simulink model "SF049A_LoaMgr"  (R2013b)
settings: Solver=FixedStepDiscrete  SolverMode=SingleTasking  StartTime=0.0  StopTime=1  FixedStep=0.002  RelTol=1e-3
undefined symbols (not defined in the file): CURRMEASLOAMTGTNMASK_CNT_U08, IVTRLOAMTGTNMASK_CNT_U08, LoaCtrldShtdwn, LoaCurrMeasIdptSigNrFlt, LoaHwTqIdptSigNrFlt, LoaImdtShtdwn, LoaIvtrIdptSigNrFlt, LOAMAXSLEW_ULSPERSEC_F32, LoaMgrCurrIvtrMtgtnRate, LoaMgrCurrIvtrMtgtnSca, LoaMgrCurrIvtrMtgtnScaZeroEna, LoaMgrCurrMeasIdptSig0Resp, LoaMgrCurrMeasIdptSig1Resp, LoaMgrCurrMeasIdptSig2Resp, LoaMgrCurrMeasIdptSigFltThd, LoaMgrCurrMeasMtgtnRate, LoaMgrCurrMeasMtgtnSca, LoaMgrCurrMeasMtgtnScaZeroEna, LoaMgrFadeOutStRate, LoaMgrHwTqIdptSig0NoTqLoaResp, LoaMgrHwTqIdptSig1NoTqLoaResp, LoaMgrHwTqIdptSig2Resp, LoaMgrHwTqIdptSig4Resp, LoaMgrHwTqIdptSigFltThd, LoaMgrHwTqLoaAvlResp, LoaMgrIvtrIdptSig0Resp, LoaMgrIvtrIdptSig1Resp, LoaMgrIvtrIdptSig2Resp, LoaMgrIvtrIdptSigFltThd, LoaMgrIvtrMtgtnRate, LoaMgrIvtrMtgtnSca, LoaMgrIvtrMtgtnScaZeroEna, LoaMgrLimdStRate, LoaMgrLimdStSca, LoaMgrMotAgAvlSnsrlsResp, LoaMgrMotAgIdptSig0NoSnsrlsResp, LoaMgrMotAgIdptSig1NoSnsrlsResp, LoaMgrMotAgIdptSig2Resp, LoaMgrMotAgIdptSig3Resp, LoaMgrMotAgIdptSigFltThd, LoaMgrMotAgMtgtnRate, LoaMgrMotAgMtgtnSca, LoaMgrMotAgMtgtnScaZeroEna, LoaMotAgIdptSigNrFlt, LOASCAONE_ULS_F32, LOASCAZERO_ULS_F32, LoaSt1, LOASTIMDTSHTDWN_CNT_U08, LOASTNORM_CNT_U08, LOASTSWMTGTN_CNT_U08, MAXCURRMEASIDPTSIGALLWD_CNT_U08, MAXHWTQIDPTSIGALLWD_CNT_U08, MAXIVTRIDPTSIGALLWD_CNT_U08, MAXMOTAGMECLIDPTSIGALLWD_CNT_U08, NODEBSTEP_CNT_U16, NtcSts1, SigQlfr1
libraries: simulink x30, NxtrMin x4, NxtrMax x4, NxtrLim x2
(part 3 of 7)

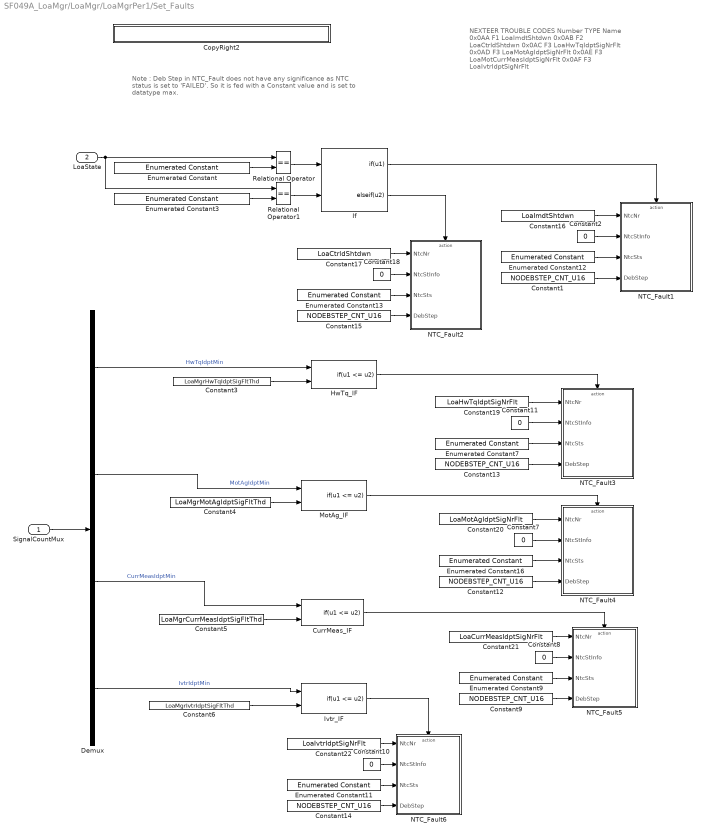
== system SF049A_LoaMgr/LoaMgr/LoaMgrPer1/Set_Faults ==
  note: Note : Deb Step in NTC_Fault does not have any significance as
      | NTC status is set to 'FAILED'. So it is fed with a Constant value and
      | is set to datatype max.
  note: NEXTEER TROUBLE CODES
      | Number  TYPE   Name
      |  0x0AA      F1      LoaImdtShtdwn
      |  0x0AB      F2      LoaCtrldShtdwn
      |  0x0AC      F3      LoaHwTqIdptSigNrFlt
      |  0x0AD      F3      LoaMotAgIdptSigNrFlt
      |  0x0AE      F3      LoaMotCurrMeasIdptSigNrFlt
      |  0x0AF      F3      LoaIvtrIdptSigNrFlt
  SignalCountMux : Inport
  LoaState : Inport  RequirementInfo={} %GIDa_be80d350_3951_4772_b695_9000f2f6daa5  Port=2
  Constant1 : Constant  RequirementInfo="{'linktype_rmi_doors' '00012fd5 (/E-STEER Core/SubSystem Specifications/Application Functions - EA4/SF049A Loss of Assist Manager)' '#SF049A_41' 'true' 'REQ:  SF049A_41' '' } %GIDa_6008ab27_f6d5_4e1f_aaef_fe9677c74400"  Value=NODEBSTEP_CNT_U16
  Constant10 : Constant  RequirementInfo="{'linktype_rmi_doors' '00012fd5 (/E-STEER Core/SubSystem Specifications/Application Functions - EA4/SF049A Loss of Assist Manager)' '#SF049A_96' 'true' 'REQ:  SF049A_96' '' } %GIDa_9d6138e1_72b7_4c86_9d87_817de0f28e02"  Value=0
  Constant11 : Constant  RequirementInfo="{'linktype_rmi_doors' '00012fd5 (/E-STEER Core/SubSystem Specifications/Application Functions - EA4/SF049A Loss of Assist Manager)' '#SF049A_63' 'true' 'REQ:  SF049A_63' '' } %GIDa_f847bbfc_c670_43d9_9c09_50e4c18d810d"  Value=0
  Constant12 : Constant  RequirementInfo="{'linktype_rmi_doors' '00012fd5 (/E-STEER Core/SubSystem Specifications/Application Functions - EA4/SF049A Loss of Assist Manager)' '#SF049A_74' 'true' 'REQ:  SF049A_74' '' } %GIDa_482641ce_f585_4632_a45d_846d40cb84bb"  Value=NODEBSTEP_CNT_U16
  Constant13 : Constant  RequirementInfo="{'linktype_rmi_doors' '00012fd5 (/E-STEER Core/SubSystem Specifications/Application Functions - EA4/SF049A Loss of Assist Manager)' '#SF049A_63' 'true' 'REQ:  SF049A_63' '' } %GIDa_516393a5_f80f_4cb2_bae9_6e4bb58c3191"  Value=NODEBSTEP_CNT_U16
  Constant14 : Constant  RequirementInfo="{'linktype_rmi_doors' '00012fd5 (/E-STEER Core/SubSystem Specifications/Application Functions - EA4/SF049A Loss of Assist Manager)' '#SF049A_96' 'true' 'REQ:  SF049A_96' '' } %GIDa_be9bb861_018d_44a6_a080_0e9c68b6dcb7"  Value=NODEBSTEP_CNT_U16
  Constant15 : Constant  RequirementInfo="{'linktype_rmi_doors' '00012fd5 (/E-STEER Core/SubSystem Specifications/Application Functions - EA4/SF049A Loss of Assist Manager)' '#SF049A_52' 'true' 'REQ:  SF049A_52' '' } %GIDa_0fe878fe_27c3_4b2a_9c4a_e08aafcb438f"  Value=NODEBSTEP_CNT_U16
  Constant16 : Constant  RequirementInfo="{'linktype_rmi_doors' '00012fd5 (/E-STEER Core/SubSystem Specifications/Application Functions - EA4/SF049A Loss of Assist Manager)' '#SF049A_41' 'true' 'REQ:  SF049A_41' '' } %GIDa_da02ad7f_2e11_4a07_a653_13476a033a59"  Value=LoaImdtShtdwn
  Constant17 : Constant  RequirementInfo="{'linktype_rmi_doors' '00012fd5 (/E-STEER Core/SubSystem Specifications/Application Functions - EA4/SF049A Loss of Assist Manager)' '#SF049A_52' 'true' 'REQ:  SF049A_52' '' } %GIDa_1c4603b7_e4a0_453d_b772_10fa4ca01a05"  Value=LoaCtrldShtdwn
  Constant18 : Constant  RequirementInfo="{'linktype_rmi_doors' '00012fd5 (/E-STEER Core/SubSystem Specifications/Application Functions - EA4/SF049A Loss of Assist Manager)' '#SF049A_52' 'true' 'REQ:  SF049A_52' '' } %GIDa_6e9baf4a_2a1d_4f2c_8c2c_bf437d4d00ad"  Value=0
  Constant19 : Constant  RequirementInfo="{'linktype_rmi_doors' '00012fd5 (/E-STEER Core/SubSystem Specifications/Application Functions - EA4/SF049A Loss of Assist Manager)' '#SF049A_63' 'true' 'REQ:  SF049A_63' '' } %GIDa_f668c260_f633_4aa9_84e3_26df089b87f3"  Value=LoaHwTqIdptSigNrFlt
  Constant2 : Constant  RequirementInfo="{'linktype_rmi_doors' '00012fd5 (/E-STEER Core/SubSystem Specifications/Application Functions - EA4/SF049A Loss of Assist Manager)' '#SF049A_41' 'true' 'REQ:  SF049A_41' '' } %GIDa_747c9c9e_ef17_47fe_b985_caf6a20fd37f"  Value=0
  Constant20 : Constant  RequirementInfo="{'linktype_rmi_doors' '00012fd5 (/E-STEER Core/SubSystem Specifications/Application Functions - EA4/SF049A Loss of Assist Manager)' '#SF049A_74' 'true' 'REQ:  SF049A_74' '' } %GIDa_14482680_3551_44f7_96ed_865902b9c606"  Value=LoaMotAgIdptSigNrFlt
  Constant21 : Constant  RequirementInfo="{'linktype_rmi_doors' '00012fd5 (/E-STEER Core/SubSystem Specifications/Application Functions - EA4/SF049A Loss of Assist Manager)' '#SF049A_85' 'true' 'REQ:  SF049A_85' '' } %GIDa_832d69b5_6fc6_4eb3_8bca_5a3f0a9135ea"  Value=LoaCurrMeasIdptSigNrFlt
  Constant22 : Constant  RequirementInfo="{'linktype_rmi_doors' '00012fd5 (/E-STEER Core/SubSystem Specifications/Application Functions - EA4/SF049A Loss of Assist Manager)' '#SF049A_96' 'true' 'REQ:  SF049A_96' '' } %GIDa_6d82d2bc_dd2c_42b2_a495_f69233371b4c"  Value=LoaIvtrIdptSigNrFlt
  Constant3 : Constant  RequirementInfo="{'linktype_rmi_doors' '00012fd5 (/E-STEER Core/SubSystem Specifications/Application Functions - EA4/SF049A Loss of Assist Manager)' '#SF049A_63' 'true' 'REQ:  SF049A_63' '' } %GIDa_37667763_620e_4899_919f_fd047f56e6a4"  Value=LoaMgrHwTqIdptSigFltThd  OutDataTypeStr=uint8
  Constant4 : Constant  RequirementInfo="{'linktype_rmi_doors' '00012fd5 (/E-STEER Core/SubSystem Specifications/Application Functions - EA4/SF049A Loss of Assist Manager)' '#SF049A_74' 'true' 'REQ:  SF049A_74' '' } %GIDa_77c93d9e_03c3_4b62_bdd1_aee578103365"  Value=LoaMgrMotAgIdptSigFltThd  OutDataTypeStr=uint8
  Constant5 : Constant  RequirementInfo="{'linktype_rmi_doors' '00012fd5 (/E-STEER Core/SubSystem Specifications/Application Functions - EA4/SF049A Loss of Assist Manager)' '#SF049A_85' 'true' 'REQ:  SF049A_85' '' } %GIDa_d64c53a0_35b8_4420_a41e_635bbd8b4ecd"  Value=LoaMgrCurrMeasIdptSigFltThd  OutDataTypeStr=uint8
  Constant6 : Constant  RequirementInfo="{'linktype_rmi_doors' '00012fd5 (/E-STEER Core/SubSystem Specifications/Application Functions - EA4/SF049A Loss of Assist Manager)' '#SF049A_96' 'true' 'REQ:  SF049A_96' '' } %GIDa_7f50743d_969b_4369_833c_68bf5c85ed87"  Value=LoaMgrIvtrIdptSigFltThd  OutDataTypeStr=uint8
  Constant7 : Constant  RequirementInfo="{'linktype_rmi_doors' '00012fd5 (/E-STEER Core/SubSystem Specifications/Application Functions - EA4/SF049A Loss of Assist Manager)' '#SF049A_74' 'true' 'REQ:  SF049A_74' '' } %GIDa_8453ac68_f225_4989_8715_19d1b6b526f1"  Value=0
  Constant8 : Constant  RequirementInfo="{'linktype_rmi_doors' '00012fd5 (/E-STEER Core/SubSystem Specifications/Application Functions - EA4/SF049A Loss of Assist Manager)' '#SF049A_85' 'true' 'REQ:  SF049A_85' '' } %GIDa_8f875e11_a213_47ed_b103_c1e7f6c8c9d1"  Value=0
  Constant9 : Constant  RequirementInfo="{'linktype_rmi_doors' '00012fd5 (/E-STEER Core/SubSystem Specifications/Application Functions - EA4/SF049A Loss of Assist Manager)' '#SF049A_85' 'true' 'REQ:  SF049A_85' '' } %GIDa_1c242d58_d7e7_407c_a342_44f914ab24c5"  Value=NODEBSTEP_CNT_U16
  CopyRight2 : Subsystem  Description=|  mask(Copyright Information){none=on}
      | Copyright info block.                                               
      |                                                                     
      | Place copyright information at the top of every subsystem in design.
      mask prompts: none "No parameters"
      mask help: Place copyright information at the top of every subsystem in design.
      mask Display:
      | NxtrConf = 'Nexteer Confidential';
      | 
      | sys = bdroot; %handle for the current model ("system")
      | first = get_param(sys,'Created');
      | first = first(end-3:end);  %year is last four digits
      | 
      | last = get_param(sys,'LastModifiedDate');
      | if isempty(last)
      |     last = datestr(now,'yyyy');
      | else
      |     last = last(end-3:end);
      | end
      | 
      | if strcmp(first,last)
      |     fprintf('%s -- Copyright %s Nexteer',NxtrConf,first)
      | else
      |     fprintf('%s -- %s%s- %s Nexteer',NxtrConf,char(169),first,last)
      | end
  CurrMeas_IF : If  RequirementInfo="{'linktype_rmi_doors' '00012fd5 (/E-STEER Core/SubSystem Specifications/Application Functions - EA4/SF049A Loss of Assist Manager)' '#SF049A_85' 'true' 'REQ:  SF049A_85' '' } %GIDa_6bfcb657_871c_41cb_8cce_44b1fe119df9"  NumInputs=2  IfExpression=u1 <= u2  ShowElse=off
  Demux : Demux
  Enumerated Constant11 : simulink/Sources/Enumerated Constant  RequirementInfo="{'linktype_rmi_doors' '00012fd5 (/E-STEER Core/SubSystem Specifications/Application Functions - EA4/SF049A Loss of Assist Manager)' '#SF049A_96' 'true' 'REQ:  SF049A_96' '' } %GIDa_713fd3e6_be26_448c_91a8_ed8494ee3c40"  OutDataTypeStr=Enum: NtcSts1  Value=NtcSts1.NTCSTS_FAILD  SampleTime=inf
  Enumerated Constant12 : simulink/Sources/Enumerated Constant  RequirementInfo="{'linktype_rmi_doors' '00012fd5 (/E-STEER Core/SubSystem Specifications/Application Functions - EA4/SF049A Loss of Assist Manager)' '#SF049A_41' 'true' 'REQ:  SF049A_41' '' } %GIDa_63ce7b73_bc20_4b35_9d10_03df4b237ddd"  OutDataTypeStr=Enum: NtcSts1  Value=NtcSts1.NTCSTS_FAILD  SampleTime=inf
  Enumerated Constant13 : simulink/Sources/Enumerated Constant  RequirementInfo="{'linktype_rmi_doors' '00012fd5 (/E-STEER Core/SubSystem Specifications/Application Functions - EA4/SF049A Loss of Assist Manager)' '#SF049A_52' 'true' 'REQ:  SF049A_52' '' } %GIDa_090eb992_316c_40d4_850d_01d1f9b0ddc1"  OutDataTypeStr=Enum: NtcSts1  Value=NtcSts1.NTCSTS_FAILD  SampleTime=inf
  Enumerated Constant16 : simulink/Sources/Enumerated Constant  RequirementInfo="{'linktype_rmi_doors' '00012fd5 (/E-STEER Core/SubSystem Specifications/Application Functions - EA4/SF049A Loss of Assist Manager)' '#SF049A_74' 'true' 'REQ:  SF049A_74' '' } %GIDa_0cbe054c_348e_4589_9d06_a6855cc600db"  OutDataTypeStr=Enum: NtcSts1  Value=NtcSts1.NTCSTS_FAILD  SampleTime=inf
  Enumerated Constant7 : simulink/Sources/Enumerated Constant  RequirementInfo="{'linktype_rmi_doors' '00012fd5 (/E-STEER Core/SubSystem Specifications/Application Functions - EA4/SF049A Loss of Assist Manager)' '#SF049A_63' 'true' 'REQ:  SF049A_63' '' } %GIDa_e7e99b92_f776_4b68_8499_db3d0ca6f8c0"  OutDataTypeStr=Enum: NtcSts1  Value=NtcSts1.NTCSTS_FAILD  SampleTime=inf
  Enumerated Constant9 : simulink/Sources/Enumerated Constant  RequirementInfo="{'linktype_rmi_doors' '00012fd5 (/E-STEER Core/SubSystem Specifications/Application Functions - EA4/SF049A Loss of Assist Manager)' '#SF049A_85' 'true' 'REQ:  SF049A_85' '' } %GIDa_061570ed_eba3_4e2b_8ec6_3a5ae72109b6"  OutDataTypeStr=Enum: NtcSts1  Value=NtcSts1.NTCSTS_FAILD  SampleTime=inf
  Enumerated Constant : simulink/Sources/Enumerated Constant  RequirementInfo="{'linktype_rmi_doors' '00012fd5 (/E-STEER Core/SubSystem Specifications/Application Functions - EA4/SF049A Loss of Assist Manager)' '#SF049A_41' 'true' 'REQ:  SF049A_41' '' } %GIDa_c587e64a_b992_420a_b427_1416918963fa"  OutDataTypeStr=Enum: LoaSt1  Value=LoaSt1.LOAST_IMDTSHTDWNREQD  SampleTime=inf
  Enumerated Constant3 : simulink/Sources/Enumerated Constant  RequirementInfo="{'linktype_rmi_doors' '00012fd5 (/E-STEER Core/SubSystem Specifications/Application Functions - EA4/SF049A Loss of Assist Manager)' '#SF049A_52' 'true' 'REQ:  SF049A_52' '' } %GIDa_26358f93_c658_49ff_84a8_2b8632a2f5dc"  OutDataTypeStr=Enum: LoaSt1  Value=LoaSt1.LOAST_CTRLDSHTDWNREQD  SampleTime=inf
  HwTq_IF : If  RequirementInfo="{'linktype_rmi_doors' '00012fd5 (/E-STEER Core/SubSystem Specifications/Application Functions - EA4/SF049A Loss of Assist Manager)' '#SF049A_63' 'true' 'REQ:  SF049A_63' '' } %GIDa_678e227d_0f84_4f14_82b0_cb31208f4dd0"  NumInputs=2  IfExpression=u1 <= u2  ShowElse=off
  If : If  RequirementInfo="{'linktype_rmi_doors' '00012fd5 (/E-STEER Core/SubSystem Specifications/Application Functions - EA4/SF049A Loss of Assist Manager)' '#SF049A_41' 'true' 'REQ:  SF049A_41' '' ; 'linktype_rmi_doors' '00012fd5 (/E-STEER Core/SubSystem Specifications/Application Functions - EA4/SF049A Loss of Assist Manager)' '#SF049A_52' 'true' 'REQ:  SF049A_52' '' } %GIDa_23c447c5_8dde_4944_ace5_375a10730015"  NumInputs=2  IfExpression=u1  ElseIfExpressions=u2  ShowElse=off
  Ivtr_IF : If  RequirementInfo="{'linktype_rmi_doors' '00012fd5 (/E-STEER Core/SubSystem Specifications/Application Functions - EA4/SF049A Loss of Assist Manager)' '#SF049A_96' 'true' 'REQ:  SF049A_96' '' } %GIDa_18461709_94ab_42e2_a069_61c0c19314cc"  NumInputs=2  IfExpression=u1 <= u2  ShowElse=off
  MotAg_IF : If  RequirementInfo="{'linktype_rmi_doors' '00012fd5 (/E-STEER Core/SubSystem Specifications/Application Functions - EA4/SF049A Loss of Assist Manager)' '#SF049A_74' 'true' 'REQ:  SF049A_74' '' } %GIDa_83f9ac87_4bd9_496c_bfc9_dd18e4d77f46"  NumInputs=2  IfExpression=u1 <= u2  ShowElse=off
  NTC_Fault1 : Subsystem  RequirementInfo="{'linktype_rmi_doors' '00012fd5 (/E-STEER Core/SubSystem Specifications/Application Functions - EA4/SF049A Loss of Assist Manager)' '#SF049A_41' 'true' 'REQ:  SF049A_41' '' } %GIDa_71298e83_2c65_4f06_9818_7aee0584e2c5"  mask(SetNTC){}
      mask help: SetNTC library block
  NTC_Fault2 : Subsystem  RequirementInfo="{'linktype_rmi_doors' '00012fd5 (/E-STEER Core/SubSystem Specifications/Application Functions - EA4/SF049A Loss of Assist Manager)' '#SF049A_52' 'true' 'REQ:  SF049A_52' '' } %GIDa_4a067bef_a03a_452c_b149_a1eda42dcd65"  mask(SetNTC){}
      mask help: SetNTC library block
  NTC_Fault3 : Subsystem  RequirementInfo="{'linktype_rmi_doors' '00012fd5 (/E-STEER Core/SubSystem Specifications/Application Functions - EA4/SF049A Loss of Assist Manager)' '#SF049A_63' 'true' 'REQ:  SF049A_63' '' } %GIDa_9a104022_4a5c_4ec3_9a4e_ff73e70c52c0"  mask(SetNTC){}
      mask help: SetNTC library block
  NTC_Fault4 : Subsystem  RequirementInfo="{'linktype_rmi_doors' '00012fd5 (/E-STEER Core/SubSystem Specifications/Application Functions - EA4/SF049A Loss of Assist Manager)' '#SF049A_74' 'true' 'REQ:  SF049A_74' '' } %GIDa_36ede392_50a1_435c_aacd_3ba31a4a699f"  mask(SetNTC){}
      mask help: SetNTC library block
  NTC_Fault5 : Subsystem  RequirementInfo="{'linktype_rmi_doors' '00012fd5 (/E-STEER Core/SubSystem Specifications/Application Functions - EA4/SF049A Loss of Assist Manager)' '#SF049A_85' 'true' 'REQ:  SF049A_85' '' } %GIDa_416c1ab8_bd82_4764_87a2_5cf35e1538c6"  mask(SetNTC){}
      mask help: SetNTC library block
  NTC_Fault6 : Subsystem  RequirementInfo="{'linktype_rmi_doors' '00012fd5 (/E-STEER Core/SubSystem Specifications/Application Functions - EA4/SF049A Loss of Assist Manager)' '#SF049A_96' 'true' 'REQ:  SF049A_96' '' } %GIDa_e4012090_43d2_4397_8c24_60789b5b70d7"  mask(SetNTC){}
      mask help: SetNTC library block
  Relational Operator : RelationalOperator  RequirementInfo="{'linktype_rmi_doors' '00012fd5 (/E-STEER Core/SubSystem Specifications/Application Functions - EA4/SF049A Loss of Assist Manager)' '#SF049A_41' 'true' 'REQ:  SF049A_41' '' } %GIDa_5b43dfc5_6961_46eb_9b6f_d0feec9657d0"  Operator===  OutDataTypeStr=boolean
  Relational Operator1 : RelationalOperator  RequirementInfo="{'linktype_rmi_doors' '00012fd5 (/E-STEER Core/SubSystem Specifications/Application Functions - EA4/SF049A Loss of Assist Manager)' '#SF049A_52' 'true' 'REQ:  SF049A_52' '' } %GIDa_73f4c8bf_5167_47bf_a964_c5c316e4a9fa"  Operator===  OutDataTypeStr=boolean
  wires:
  Constant13/1 -> NTC_Fault3/4(DebStep)
  Enumerated Constant7/1 -> NTC_Fault3/3(NtcSts)
  Constant11/1 -> NTC_Fault3/2(NtcStInfo)
  Constant19/1 -> NTC_Fault3/1(NtcNr)
  Constant12/1 -> NTC_Fault4/4(DebStep)
  Enumerated Constant16/1 -> NTC_Fault4/3(NtcSts)
  Constant7/1 -> NTC_Fault4/2(NtcStInfo)
  Constant20/1 -> NTC_Fault4/1(NtcNr)
  Constant1/1 -> NTC_Fault1/4(DebStep)
  Enumerated Constant12/1 -> NTC_Fault1/3(NtcSts)
  Constant2/1 -> NTC_Fault1/2(NtcStInfo)
  Constant16/1 -> NTC_Fault1/1(NtcNr)
  Constant17/1 -> NTC_Fault2/1(NtcNr)
  Constant18/1 -> NTC_Fault2/2(NtcStInfo)
  Enumerated Constant13/1 -> NTC_Fault2/3(NtcSts)
  Constant15/1 -> NTC_Fault2/4(DebStep)
  Ivtr_IF/1 -> NTC_Fault6/Action
  Constant14/1 -> NTC_Fault6/4(DebStep)
  Enumerated Constant11/1 -> NTC_Fault6/3(NtcSts)
  Constant10/1 -> NTC_Fault6/2(NtcStInfo)
  Constant22/1 -> NTC_Fault6/1(NtcNr)
  CurrMeas_IF/1 -> NTC_Fault5/Action
  Constant9/1 -> NTC_Fault5/4(DebStep)
  Enumerated Constant9/1 -> NTC_Fault5/3(NtcSts)
  Constant8/1 -> NTC_Fault5/2(NtcStInfo)
  Constant21/1 -> NTC_Fault5/1(NtcNr)
  MotAg_IF/1 -> NTC_Fault4/Action
  HwTq_IF/1 -> NTC_Fault3/Action
  Demux/4 -> Ivtr_IF/1  "IvtrIdptMin"
  Constant6/1 -> Ivtr_IF/2
  Demux/3 -> CurrMeas_IF/1  "CurrMeasIdptMin"
  Constant5/1 -> CurrMeas_IF/2
  Demux/2 -> MotAg_IF/1  "MotAgIdptMin"
  Constant4/1 -> MotAg_IF/2
  Demux/1 -> HwTq_IF/1  "HwTqIdptMin"
  Constant3/1 -> HwTq_IF/2
  SignalCountMux/1 -> Demux/1
  Relational Operator/1 -> If/1
  Relational Operator1/1 -> If/2
  LoaState/1 -> Relational Operator1/1, Relational Operator/1
  Enumerated Constant3/1 -> Relational Operator1/2
  Enumerated Constant/1 -> Relational Operator/2
  If/1 -> NTC_Fault1/Action
  If/2 -> NTC_Fault2/Action

== system SF049A_LoaMgr/LoaMgr/LoaMgrPer1/else ==
  In1 : Inport
  Action Port : ActionPort  ActionType=else
  Out1 : Outport
  wires:
  In1/1 -> Out1/1

== system SF049A_LoaMgr/LoaMgr/LoaMgrPer1/if ==
  Action Port : ActionPort  ActionType=then
  Constant : Constant  OutDataTypeStr=Inherit: Inherit via back propagation
  Out1 : Outport
  wires:
  Constant/1 -> Out1/1

== system SF049A_LoaMgr/ISO Fault Debounce/DiagMgr/NTCSTS_PREFAILD/CopyRight2 ==

== system SF049A_LoaMgr/ISO Fault Debounce/DiagMgr/NTCSTS_PREFAILD/If Action Subsystem ==
  DS : Inport
  Qlf : Inport  Port=2
  Action Port : ActionPort  ActionType=then
  EAo : Outport
  Qlfo : Outport  Port=2
  wires:
  Qlf/1 -> Qlfo/1
  DS/1 -> EAo/1

== system SF049A_LoaMgr/ISO Fault Debounce/DiagMgr/NTCSTS_PREFAILD/If Action Subsystem1 ==
  DS : Inport
  EA : Inport  Port=2
  Qlf : Inport  Port=3
  TS : Inport  Port=4
  Action Port : ActionPort  ActionType=else
  CopyRight2 : Subsystem  Description=|  mask(Copyright Information){none=on}
      | Copyright info block.                                               
      |                                                                     
      | Place copyright information at the top of every subsystem in design.
      mask prompts: none "No parameters"
      mask help: Place copyright information at the top of every subsystem in design.
      mask Display:
      | NxtrConf = 'Nexteer Confidential';
      | 
      | sys = bdroot; %handle for the current model ("system")
      | first = get_param(sys,'Created');
      | first = first(end-3:end);  %year is last four digits
      | 
      | last = get_param(sys,'LastModifiedDate');
      | if isempty(last)
      |     last = datestr(now,'yyyy');
      | else
      |     last = last(end-3:end);
      | end
      | 
      | if strcmp(first,last)
      |     fprintf('%s -- Copyright %s Nexteer',NxtrConf,first)
      | else
      |     fprintf('%s -- %s%s- %s Nexteer',NxtrConf,char(169),first,last)
      | end
  If : If  NumInputs=2  IfExpression=u1 < u2
  If Action Subsystem : Subsystem  TreatAsAtomicUnit=on
  If Action Subsystem1 : Subsystem  TreatAsAtomicUnit=on
  Merge : Merge
  Merge1 : Merge
  QFFailed : Constant  Value=SigQlfr1.SIGQLFR_FAILD  OutDataTypeStr=Enum: SigQlfr1
  Sum : Sum  Inputs=|++
  EAo : Outport
  Qlfo : Outport  Port=2
  wires:
  DS/1 -> Sum/1
  EA/1 -> Sum/2
  Sum/1 -> If Action Subsystem/1(EA), If/1
  TS/1 -> If Action Subsystem1/1(EA), If/2
  If/2 -> If Action Subsystem1/Action
  If/1 -> If Action Subsystem/Action
  Qlf/1 -> If Action Subsystem/2(Qlf)
  QFFailed/1 -> If Action Subsystem1/2(Qlf)
  Merge1/1 -> Qlfo/1
  Merge/1 -> EAo/1
  If Action Subsystem1/1(EAo) -> Merge/1
  If Action Subsystem/1(EAo) -> Merge/2
  If Action Subsystem1/2(Qlfo) -> Merge1/1
  If Action Subsystem/2(Qlfo) -> Merge1/2

== system SF049A_LoaMgr/ISO Fault Debounce/DiagMgr/NTCSTS_PREPASSD/CopyRight2 ==

== system SF049A_LoaMgr/ISO Fault Debounce/DiagMgr/NTCSTS_PREPASSD/If Action Subsystem ==
  In1 : Inport
  In2 : Inport  Port=2
  Action Port : ActionPort  ActionType=then
  Out1 : Outport
  Out2 : Outport  Port=2
  wires:
  In1/1 -> Out1/1
  In2/1 -> Out2/1

== system SF049A_LoaMgr/ISO Fault Debounce/DiagMgr/NTCSTS_PREPASSD/If Action Subsystem1 ==
  In1 : Inport
  In2 : Inport  Port=2
  Action Port : ActionPort  ActionType=else
  Out1 : Outport
  Out2 : Outport  Port=2
  wires:
  In1/1 -> Out1/1
  In2/1 -> Out2/1

== system SF049A_LoaMgr/LoaMgr/LoaMgrInit1/NTC_Fault1/SetNtcSts ==
  NtcNr : Inport
  NtcStInfo : Inport  Port=2
  NtcSts : Inport  Port=3
  DebStep : Inport  Port=4
  CopyRight2 : Subsystem  Description=|  mask(Copyright Information){none=on}
      | Copyright info block.                                               
      |                                                                     
      | Place copyright information at the top of every subsystem in design.
      mask prompts: none "No parameters"
      mask help: Place copyright information at the top of every subsystem in design.
      mask Display:
      | NxtrConf = 'Nexteer Confidential';
      | 
      | sys = bdroot; %handle for the current model ("system")
      | first = get_param(sys,'Created');
      | first = first(end-3:end);  %year is last four digits
      | 
      | last = get_param(sys,'LastModifiedDate');
      | if isempty(last)
      |     last = datestr(now,'yyyy');
      | else
      |     last = last(end-3:end);
      | end
      | 
      | if strcmp(first,last)
      |     fprintf('%s -- Copyright %s Nexteer',NxtrConf,first)
      | else
      |     fprintf('%s -- %s%s- %s Nexteer',NxtrConf,char(169),first,last)
      | end
  Data Store Write1 : DataStoreWrite  DataStoreName=DebStep
  Data Store Write3 : DataStoreWrite  DataStoreName=Fault1_Status
  Terminator : Terminator
  Terminator1 : Terminator
  wires:
  DebStep/1 -> Data Store Write1/1
  NtcSts/1 -> Data Store Write3/1
  NtcNr/1 -> Terminator/1
  NtcStInfo/1 -> Terminator1/1

== system SF049A_LoaMgr/LoaMgr/LoaMgrInit1/NTC_Fault2/SetNtcSts ==
  NtcNr : Inport
  NtcStInfo : Inport  Port=2
  NtcSts : Inport  Port=3
  DebStep : Inport  Port=4
  CopyRight2 : Subsystem  Description=|  mask(Copyright Information){none=on}
      | Copyright info block.                                               
      |                                                                     
      | Place copyright information at the top of every subsystem in design.
      mask prompts: none "No parameters"
      mask help: Place copyright information at the top of every subsystem in design.
      mask Display:
      | NxtrConf = 'Nexteer Confidential';
      | 
      | sys = bdroot; %handle for the current model ("system")
      | first = get_param(sys,'Created');
      | first = first(end-3:end);  %year is last four digits
      | 
      | last = get_param(sys,'LastModifiedDate');
      | if isempty(last)
      |     last = datestr(now,'yyyy');
      | else
      |     last = last(end-3:end);
      | end
      | 
      | if strcmp(first,last)
      |     fprintf('%s -- Copyright %s Nexteer',NxtrConf,first)
      | else
      |     fprintf('%s -- %s%s- %s Nexteer',NxtrConf,char(169),first,last)
      | end
  Data Store Write1 : DataStoreWrite  DataStoreName=DebStep
  Data Store Write3 : DataStoreWrite  DataStoreName=Fault2_Status
  Terminator : Terminator
  Terminator1 : Terminator
  wires:
  NtcStInfo/1 -> Terminator1/1
  NtcNr/1 -> Terminator/1
  NtcSts/1 -> Data Store Write3/1
  DebStep/1 -> Data Store Write1/1

== system SF049A_LoaMgr/LoaMgr/LoaMgrInit1/NTC_Fault3/SetNtcSts ==
  NtcNr : Inport
  NtcStInfo : Inport  Port=2
  NtcSts : Inport  Port=3
  DebStep : Inport  Port=4
  CopyRight2 : Subsystem  Description=|  mask(Copyright Information){none=on}
      | Copyright info block.                                               
      |                                                                     
      | Place copyright information at the top of every subsystem in design.
      mask prompts: none "No parameters"
      mask help: Place copyright information at the top of every subsystem in design.
      mask Display:
      | NxtrConf = 'Nexteer Confidential';
      | 
      | sys = bdroot; %handle for the current model ("system")
      | first = get_param(sys,'Created');
      | first = first(end-3:end);  %year is last four digits
      | 
      | last = get_param(sys,'LastModifiedDate');
      | if isempty(last)
      |     last = datestr(now,'yyyy');
      | else
      |     last = last(end-3:end);
      | end
      | 
      | if strcmp(first,last)
      |     fprintf('%s -- Copyright %s Nexteer',NxtrConf,first)
      | else
      |     fprintf('%s -- %s%s- %s Nexteer',NxtrConf,char(169),first,last)
      | end
  Data Store Write1 : DataStoreWrite  DataStoreName=DebStep
  Data Store Write3 : DataStoreWrite  DataStoreName=Fault3_Status
  Terminator : Terminator
  Terminator1 : Terminator
  wires:
  NtcStInfo/1 -> Terminator1/1
  NtcNr/1 -> Terminator/1
  NtcSts/1 -> Data Store Write3/1
  DebStep/1 -> Data Store Write1/1

== system SF049A_LoaMgr/LoaMgr/LoaMgrInit1/NTC_Fault4/SetNtcSts ==
  NtcNr : Inport
  NtcStInfo : Inport  Port=2
  NtcSts : Inport  Port=3
  DebStep : Inport  Port=4
  CopyRight2 : Subsystem  Description=|  mask(Copyright Information){none=on}
      | Copyright info block.                                               
      |                                                                     
      | Place copyright information at the top of every subsystem in design.
      mask prompts: none "No parameters"
      mask help: Place copyright information at the top of every subsystem in design.
      mask Display:
      | NxtrConf = 'Nexteer Confidential';
      | 
      | sys = bdroot; %handle for the current model ("system")
      | first = get_param(sys,'Created');
      | first = first(end-3:end);  %year is last four digits
      | 
      | last = get_param(sys,'LastModifiedDate');
      | if isempty(last)
      |     last = datestr(now,'yyyy');
      | else
      |     last = last(end-3:end);
      | end
      | 
      | if strcmp(first,last)
      |     fprintf('%s -- Copyright %s Nexteer',NxtrConf,first)
      | else
      |     fprintf('%s -- %s%s- %s Nexteer',NxtrConf,char(169),first,last)
      | end
  Data Store Write1 : DataStoreWrite  DataStoreName=DebStep
  Data Store Write3 : DataStoreWrite  DataStoreName=Fault4_Status
  Terminator : Terminator
  Terminator1 : Terminator
  wires:
  DebStep/1 -> Data Store Write1/1
  NtcSts/1 -> Data Store Write3/1
  NtcNr/1 -> Terminator/1
  NtcStInfo/1 -> Terminator1/1

== system SF049A_LoaMgr/LoaMgr/LoaMgrInit1/NTC_Fault5/SetNtcSts ==
  NtcNr : Inport
  NtcStInfo : Inport  Port=2
  NtcSts : Inport  Port=3
  DebStep : Inport  Port=4
  CopyRight2 : Subsystem  Description=|  mask(Copyright Information){none=on}
      | Copyright info block.                                               
      |                                                                     
      | Place copyright information at the top of every subsystem in design.
      mask prompts: none "No parameters"
      mask help: Place copyright information at the top of every subsystem in design.
      mask Display:
      | NxtrConf = 'Nexteer Confidential';
      | 
      | sys = bdroot; %handle for the current model ("system")
      | first = get_param(sys,'Created');
      | first = first(end-3:end);  %year is last four digits
      | 
      | last = get_param(sys,'LastModifiedDate');
      | if isempty(last)
      |     last = datestr(now,'yyyy');
      | else
      |     last = last(end-3:end);
      | end
      | 
      | if strcmp(first,last)
      |     fprintf('%s -- Copyright %s Nexteer',NxtrConf,first)
      | else
      |     fprintf('%s -- %s%s- %s Nexteer',NxtrConf,char(169),first,last)
      | end
  Data Store Write1 : DataStoreWrite  DataStoreName=DebStep
  Data Store Write3 : DataStoreWrite  DataStoreName=Fault5_Status
  Terminator : Terminator
  Terminator1 : Terminator
  wires:
  NtcStInfo/1 -> Terminator1/1
  NtcNr/1 -> Terminator/1
  NtcSts/1 -> Data Store Write3/1
  DebStep/1 -> Data Store Write1/1

== system SF049A_LoaMgr/LoaMgr/LoaMgrInit1/NTC_Fault6/SetNtcSts ==
  NtcNr : Inport
  NtcStInfo : Inport  Port=2
  NtcSts : Inport  Port=3
  DebStep : Inport  Port=4
  CopyRight2 : Subsystem  Description=|  mask(Copyright Information){none=on}
      | Copyright info block.                                               
      |                                                                     
      | Place copyright information at the top of every subsystem in design.
      mask prompts: none "No parameters"
      mask help: Place copyright information at the top of every subsystem in design.
      mask Display:
      | NxtrConf = 'Nexteer Confidential';
      | 
      | sys = bdroot; %handle for the current model ("system")
      | first = get_param(sys,'Created');
      | first = first(end-3:end);  %year is last four digits
      | 
      | last = get_param(sys,'LastModifiedDate');
      | if isempty(last)
      |     last = datestr(now,'yyyy');
      | else
      |     last = last(end-3:end);
      | end
      | 
      | if strcmp(first,last)
      |     fprintf('%s -- Copyright %s Nexteer',NxtrConf,first)
      | else
      |     fprintf('%s -- %s%s- %s Nexteer',NxtrConf,char(169),first,last)
      | end
  Data Store Write1 : DataStoreWrite  DataStoreName=DebStep
  Data Store Write3 : DataStoreWrite  DataStoreName=Fault6_Status
  Terminator : Terminator
  Terminator1 : Terminator
  wires:
  NtcStInfo/1 -> Terminator1/1
  NtcNr/1 -> Terminator/1
  NtcSts/1 -> Data Store Write3/1
  DebStep/1 -> Data Store Write1/1

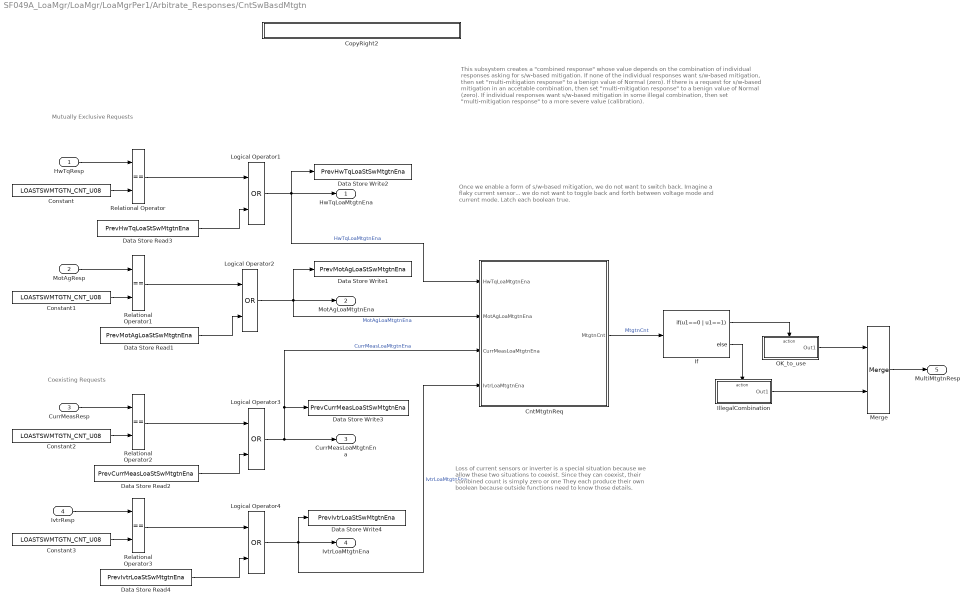
== system SF049A_LoaMgr/LoaMgr/LoaMgrPer1/Arbitrate_Responses/CntSwBasdMtgtn ==
  note: Loss of current sensors or inverter is a special situation because
      | we allow these two situations to coexist.  Since they can coexist,
      | their combined count is simply zero or one
      |
      | They each produce their own boolean because outside functions
      | need to know those details.
  note: Once we enable a form of s/w-based mitigation, we do not want to switch back.  Imagine
      | a flaky current sensor... we do not want to toggle back and forth between voltage mode
      | and current mode.  Latch each boolean true.
  note: This subsystem creates a "combined response" whose value depends on the combination of individual responses asking for s/w-based mitigation.
      |    If none of the individual responses want s/w-based mitigation,                          then set "multi-mitigation response" to a benign value of Normal (zero).
      |    If there is a request for s/w-based mitigation in an accetable combination,        then set "multi-mitigation response" to a benign value of Normal (zero).
      |    If individual responses want s/w-based mitigation in some illegal combination, then set "multi-mitigation response" to a more severe value (calibration).
  note: Mutually Exclusive Requests
  note: Coexisting Requests
  HwTqResp : Inport  RequirementInfo="{'linktype_rmi_doors' '00012fd5 (/E-STEER Core/SubSystem Specifications/Application Functions - EA4/SF049A Loss of Assist Manager)' '#SF049A_132' 'true' 'REQ:  SF049A_132' '' } %GIDa_973658ba_a4f2_4d9a_a770_f52556e4f22c"
  MotAgResp : Inport  RequirementInfo="{'linktype_rmi_doors' '00012fd5 (/E-STEER Core/SubSystem Specifications/Application Functions - EA4/SF049A Loss of Assist Manager)' '#SF049A_133' 'true' 'REQ:  SF049A_133' '' } %GIDa_aeef65fd_49ec_4123_90ed_7d409f014b7e"  Port=2
  CurrMeasResp : Inport  RequirementInfo="{'linktype_rmi_doors' '00012fd5 (/E-STEER Core/SubSystem Specifications/Application Functions - EA4/SF049A Loss of Assist Manager)' '#SF049A_134' 'true' 'REQ:  SF049A_134' '' } %GIDa_87b8fedb_e4ba_46bf_91a3_f11dc22481c0"  Port=3
  IvtrResp : Inport  RequirementInfo="{'linktype_rmi_doors' '00012fd5 (/E-STEER Core/SubSystem Specifications/Application Functions - EA4/SF049A Loss of Assist Manager)' '#SF049A_135' 'true' 'REQ:  SF049A_135' '' } %GIDa_345d2624_d4d4_491b_bfcf_9cda6a5d6213"  Port=4
  CntMtgtnReq : Subsystem
  Constant : Constant  RequirementInfo="{'linktype_rmi_doors' '00012fd5 (/E-STEER Core/SubSystem Specifications/Application Functions - EA4/SF049A Loss of Assist Manager)' '#SF049A_132' 'true' 'REQ:  SF049A_132' '' } %GIDa_418a8670_608d_4e6e_8827_6f20d11d099c"  Value=LOASTSWMTGTN_CNT_U08
  Constant1 : Constant  RequirementInfo="{'linktype_rmi_doors' '00012fd5 (/E-STEER Core/SubSystem Specifications/Application Functions - EA4/SF049A Loss of Assist Manager)' '#SF049A_133' 'true' 'REQ:  SF049A_133' '' } %GIDa_6b745ac5_2bbc_497a_ae65_5feaf681069c"  Value=LOASTSWMTGTN_CNT_U08
  Constant2 : Constant  RequirementInfo="{'linktype_rmi_doors' '00012fd5 (/E-STEER Core/SubSystem Specifications/Application Functions - EA4/SF049A Loss of Assist Manager)' '#SF049A_134' 'true' 'REQ:  SF049A_134' '' } %GIDa_687f0216_3c62_4dcd_b95a_023f5b18f54d"  Value=LOASTSWMTGTN_CNT_U08
  Constant3 : Constant  RequirementInfo="{'linktype_rmi_doors' '00012fd5 (/E-STEER Core/SubSystem Specifications/Application Functions - EA4/SF049A Loss of Assist Manager)' '#SF049A_135' 'true' 'REQ:  SF049A_135' '' } %GIDa_f7b8d234_4bac_4494_af88_077153fd1fbe"  Value=LOASTSWMTGTN_CNT_U08
  CopyRight2 : Subsystem  Description=|  mask(Copyright Information){none=on}
      | Copyright info block.                                               
      |                                                                     
      | Place copyright information at the top of every subsystem in design.
      mask prompts: none "No parameters"
      mask help: Place copyright information at the top of every subsystem in design.
      mask Display:
      | NxtrConf = 'Nexteer Confidential';
      | 
      | sys = bdroot; %handle for the current model ("system")
      | first = get_param(sys,'Created');
      | first = first(end-3:end);  %year is last four digits
      | 
      | last = get_param(sys,'LastModifiedDate');
      | if isempty(last)
      |     last = datestr(now,'yyyy');
      | else
      |     last = last(end-3:end);
      | end
      | 
      | if strcmp(first,last)
      |     fprintf('%s -- Copyright %s Nexteer',NxtrConf,first)
      | else
      |     fprintf('%s -- %s%s- %s Nexteer',NxtrConf,char(169),first,last)
      | end
  Data Store Read1 : DataStoreRead  RequirementInfo="{'linktype_rmi_doors' '00012fd5 (/E-STEER Core/SubSystem Specifications/Application Functions - EA4/SF049A Loss of Assist Manager)' '#SF049A_133' 'true' 'REQ:  SF049A_133' '' } %GIDa_436fbea6_2333_4f6b_b03d_55027604f08b"  DataStoreName=PrevMotAgLoaStSwMtgtnEna
  Data Store Read2 : DataStoreRead  RequirementInfo="{'linktype_rmi_doors' '00012fd5 (/E-STEER Core/SubSystem Specifications/Application Functions - EA4/SF049A Loss of Assist Manager)' '#SF049A_134' 'true' 'REQ:  SF049A_134' '' } %GIDa_cfb6f837_587f_40c4_be3d_46376f9b418e"  DataStoreName=PrevCurrMeasLoaStSwMtgtnEna
  Data Store Read3 : DataStoreRead  RequirementInfo="{'linktype_rmi_doors' '00012fd5 (/E-STEER Core/SubSystem Specifications/Application Functions - EA4/SF049A Loss of Assist Manager)' '#SF049A_132' 'true' 'REQ:  SF049A_132' '' } %GIDa_f6177534_403f_450f_b6ac_7b61ae77b4af"  DataStoreName=PrevHwTqLoaStSwMtgtnEna
  Data Store Read4 : DataStoreRead  RequirementInfo="{'linktype_rmi_doors' '00012fd5 (/E-STEER Core/SubSystem Specifications/Application Functions - EA4/SF049A Loss of Assist Manager)' '#SF049A_135' 'true' 'REQ:  SF049A_135' '' } %GIDa_6bdd7d0d_d1d1_46c1_a573_0ac716c4f028"  DataStoreName=PrevIvtrLoaStSwMtgtnEna
  Data Store Write1 : DataStoreWrite  RequirementInfo="{'linktype_rmi_doors' '00012fd5 (/E-STEER Core/SubSystem Specifications/Application Functions - EA4/SF049A Loss of Assist Manager)' '#SF049A_133' 'true' 'REQ:  SF049A_133' '' } %GIDa_4f65d360_a76b_4fa5_9807_6afab77b9040"  DataStoreName=PrevMotAgLoaStSwMtgtnEna
  Data Store Write2 : DataStoreWrite  RequirementInfo="{'linktype_rmi_doors' '00012fd5 (/E-STEER Core/SubSystem Specifications/Application Functions - EA4/SF049A Loss of Assist Manager)' '#SF049A_132' 'true' 'REQ:  SF049A_132' '' } %GIDa_f57a6274_f1bd_4509_a92d_2cae8afa9d2c"  DataStoreName=PrevHwTqLoaStSwMtgtnEna
  Data Store Write3 : DataStoreWrite  RequirementInfo="{'linktype_rmi_doors' '00012fd5 (/E-STEER Core/SubSystem Specifications/Application Functions - EA4/SF049A Loss of Assist Manager)' '#SF049A_134' 'true' 'REQ:  SF049A_134' '' } %GIDa_0d940290_aaa9_498b_9600_3852aeae39af"  DataStoreName=PrevCurrMeasLoaStSwMtgtnEna
  Data Store Write4 : DataStoreWrite  RequirementInfo="{'linktype_rmi_doors' '00012fd5 (/E-STEER Core/SubSystem Specifications/Application Functions - EA4/SF049A Loss of Assist Manager)' '#SF049A_135' 'true' 'REQ:  SF049A_135' '' } %GIDa_b3ee65c8_b3c0_4cba_9e64_e976312123ff"  DataStoreName=PrevIvtrLoaStSwMtgtnEna
  If : If  RequirementInfo="{'linktype_rmi_doors' '00012fd5 (/E-STEER Core/SubSystem Specifications/Application Functions - EA4/SF049A Loss of Assist Manager)' '#SF049A_143' 'true' 'REQ:  SF049A_143' '' ; 'linktype_rmi_doors' '00012fd5 (/E-STEER Core/SubSystem Specifications/Application Functions - EA4/SF049A Loss of Assist Manager)' '#SF049A_144' 'true' 'REQ:  SF049A_144' '' } %GIDa_fda17a6a_d8e3_4952_bcd8_7f6e9dbce51e"  IfExpression=u1==0 | u1==1
  IllegalCombination : Subsystem  RequirementInfo="{'linktype_rmi_doors' '00012fd5 (/E-STEER Core/SubSystem Specifications/Application Functions - EA4/SF049A Loss of Assist Manager)' '#SF049A_144' 'true' 'REQ:  SF049A_144' '' } %GIDa_1c0f47fd_321d_45b4_9de6_8e2d0dad62b4"  TreatAsAtomicUnit=on
  Logical Operator1 : Logic  RequirementInfo="{'linktype_rmi_doors' '00012fd5 (/E-STEER Core/SubSystem Specifications/Application Functions - EA4/SF049A Loss of Assist Manager)' '#SF049A_132' 'true' 'REQ:  SF049A_132' '' } %GIDa_f2dfcc8f_1474_46fe_af61_0f942cd5b2bb"  Operator=OR  AllPortsSameDT=off  OutDataTypeStr=boolean
  Logical Operator2 : Logic  RequirementInfo="{'linktype_rmi_doors' '00012fd5 (/E-STEER Core/SubSystem Specifications/Application Functions - EA4/SF049A Loss of Assist Manager)' '#SF049A_133' 'true' 'REQ:  SF049A_133' '' } %GIDa_c2a31aaa_e586_4e94_825f_4c1f2ffa4e16"  Operator=OR  AllPortsSameDT=off  OutDataTypeStr=boolean
  Logical Operator3 : Logic  RequirementInfo="{'linktype_rmi_doors' '00012fd5 (/E-STEER Core/SubSystem Specifications/Application Functions - EA4/SF049A Loss of Assist Manager)' '#SF049A_134' 'true' 'REQ:  SF049A_134' '' } %GIDa_774ae82b_4f19_4e83_aeae_dc8e846963de"  Operator=OR  AllPortsSameDT=off  OutDataTypeStr=boolean
  Logical Operator4 : Logic  RequirementInfo="{'linktype_rmi_doors' '00012fd5 (/E-STEER Core/SubSystem Specifications/Application Functions - EA4/SF049A Loss of Assist Manager)' '#SF049A_135' 'true' 'REQ:  SF049A_135' '' } %GIDa_50a49337_acd6_4944_9016_f3965f30cb79"  Operator=OR  AllPortsSameDT=off  OutDataTypeStr=boolean
  Merge : Merge  RequirementInfo="{'linktype_rmi_doors' '00012fd5 (/E-STEER Core/SubSystem Specifications/Application Functions - EA4/SF049A Loss of Assist Manager)' '#SF049A_143' 'true' 'REQ:  SF049A_143' '' ; 'linktype_rmi_doors' '00012fd5 (/E-STEER Core/SubSystem Specifications/Application Functions - EA4/SF049A Loss of Assist Manager)' '#SF049A_144' 'true' 'REQ:  SF049A_144' '' } %GIDa_3e1e40ae_b498_461c_98ff_e17942487fc6"
  OK_to_use : Subsystem  RequirementInfo="{'linktype_rmi_doors' '00012fd5 (/E-STEER Core/SubSystem Specifications/Application Functions - EA4/SF049A Loss of Assist Manager)' '#SF049A_143' 'true' 'REQ:  SF049A_143' '' } %GIDa_3d184ab3_70dc_45d4_be5c_438260c53cdd"  TreatAsAtomicUnit=on
  Relational Operator : RelationalOperator  RequirementInfo="{'linktype_rmi_doors' '00012fd5 (/E-STEER Core/SubSystem Specifications/Application Functions - EA4/SF049A Loss of Assist Manager)' '#SF049A_132' 'true' 'REQ:  SF049A_132' '' } %GIDa_92d1a1f4_8539_44a7_a24e_e34b88d9655d"  Operator===  OutDataTypeStr=boolean
  Relational Operator1 : RelationalOperator  RequirementInfo="{'linktype_rmi_doors' '00012fd5 (/E-STEER Core/SubSystem Specifications/Application Functions - EA4/SF049A Loss of Assist Manager)' '#SF049A_133' 'true' 'REQ:  SF049A_133' '' } %GIDa_625ffa2c_2126_4d8e_bf2e_a42de9ff5ff4"  Operator===  OutDataTypeStr=boolean
  Relational Operator2 : RelationalOperator  RequirementInfo="{'linktype_rmi_doors' '00012fd5 (/E-STEER Core/SubSystem Specifications/Application Functions - EA4/SF049A Loss of Assist Manager)' '#SF049A_134' 'true' 'REQ:  SF049A_134' '' } %GIDa_5dca5426_d9eb_4d6a_aebb_a973ec2043d6"  Operator===  OutDataTypeStr=boolean
  Relational Operator3 : RelationalOperator  RequirementInfo="{'linktype_rmi_doors' '00012fd5 (/E-STEER Core/SubSystem Specifications/Application Functions - EA4/SF049A Loss of Assist Manager)' '#SF049A_135' 'true' 'REQ:  SF049A_135' '' } %GIDa_0f279163_dd96_4747_9c17_108ee5b73ce7"  Operator===  OutDataTypeStr=boolean
  HwTqLoaMtgtnEna : Outport  RequirementInfo="{'linktype_rmi_doors' '00012fd5 (/E-STEER Core/SubSystem Specifications/Application Functions - EA4/SF049A Loss of Assist Manager)' '#SF049A_132' 'true' 'REQ:  SF049A_132' '' } %GIDa_90a5b576_2445_47d0_8288_42b726c3b5ea"
  MotAgLoaMtgtnEna : Outport  RequirementInfo="{'linktype_rmi_doors' '00012fd5 (/E-STEER Core/SubSystem Specifications/Application Functions - EA4/SF049A Loss of Assist Manager)' '#SF049A_133' 'true' 'REQ:  SF049A_133' '' } %GIDa_c227eae6_b027_4d1a_a0de_c29dc80723e0"  Port=2
  CurrMeasLoaMtgtnEna : Outport  RequirementInfo="{'linktype_rmi_doors' '00012fd5 (/E-STEER Core/SubSystem Specifications/Application Functions - EA4/SF049A Loss of Assist Manager)' '#SF049A_134' 'true' 'REQ:  SF049A_134' '' } %GIDa_e5f48ee4_437c_45e4_90ba_ef700f138d09"  Port=3
  IvtrLoaMtgtnEna : Outport  RequirementInfo="{'linktype_rmi_doors' '00012fd5 (/E-STEER Core/SubSystem Specifications/Application Functions - EA4/SF049A Loss of Assist Manager)' '#SF049A_135' 'true' 'REQ:  SF049A_135' '' } %GIDa_6cb87dbf_54e9_40dc_b5c0_114c9507c1bd"  Port=4
  MultiMtgtnResp : Outport  RequirementInfo={} %GIDa_62a3067c_8f3a_416f_af7f_427e2b3e6292  Port=5
  wires:
  Merge/1 -> MultiMtgtnResp/1
  IllegalCombination/1(Out1) -> Merge/2
  OK_to_use/1(Out1) -> Merge/1
  If/2 -> IllegalCombination/Action
  If/1 -> OK_to_use/Action
  CntMtgtnReq/1(MtgtnCnt) -> If/1  "MtgtnCnt"
  Data Store Read4/1 -> Logical Operator4/2
  Logical Operator4/1 -> IvtrLoaMtgtnEna/1, CntMtgtnReq/4(IvtrLoaMtgtnEna), Data Store Write4/1  "IvtrLoaMtgtnEna"
  Relational Operator3/1 -> Logical Operator4/1
  Constant3/1 -> Relational Operator3/2
  IvtrResp/1 -> Relational Operator3/1
  Data Store Read2/1 -> Logical Operator3/2
  Logical Operator3/1 -> CntMtgtnReq/3(CurrMeasLoaMtgtnEna), Data Store Write3/1, CurrMeasLoaMtgtnEna/1  "CurrMeasLoaMtgtnEna"
  Relational Operator2/1 -> Logical Operator3/1
  Constant2/1 -> Relational Operator2/2
  CurrMeasResp/1 -> Relational Operator2/1
  Data Store Read1/1 -> Logical Operator2/2
  Logical Operator2/1 -> Data Store Write1/1, CntMtgtnReq/2(MotAgLoaMtgtnEna), MotAgLoaMtgtnEna/1  "MotAgLoaMtgtnEna"
  Relational Operator1/1 -> Logical Operator2/1
  Constant1/1 -> Relational Operator1/2
  MotAgResp/1 -> Relational Operator1/1
  Data Store Read3/1 -> Logical Operator1/2
  Logical Operator1/1 -> HwTqLoaMtgtnEna/1, CntMtgtnReq/1(HwTqLoaMtgtnEna), Data Store Write2/1  "HwTqLoaMtgtnEna"
  Relational Operator/1 -> Logical Operator1/1
  Constant/1 -> Relational Operator/2
  HwTqResp/1 -> Relational Operator/1

== system SF049A_LoaMgr/LoaMgr/LoaMgrPer1/Arbitrate_Responses/CopyRight2 ==
